simulink model "EqualizerSimulinkModel"  (R2025b)
settings: Solver=VariableStepAuto  StartTime=0.0  StopTime=10.0  RelTol=1e-3
undefined symbols (not defined in the file): dspblkCoreblockFVToolHelper, gcbh
libraries: simulink x5, dspvision x1

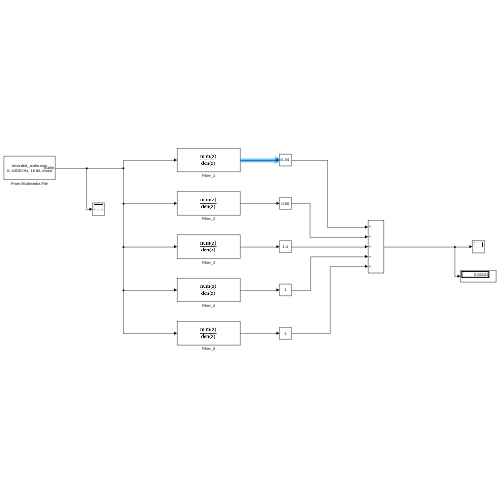
[thumbnail: Simulink's stored preview of the top-level diagram]
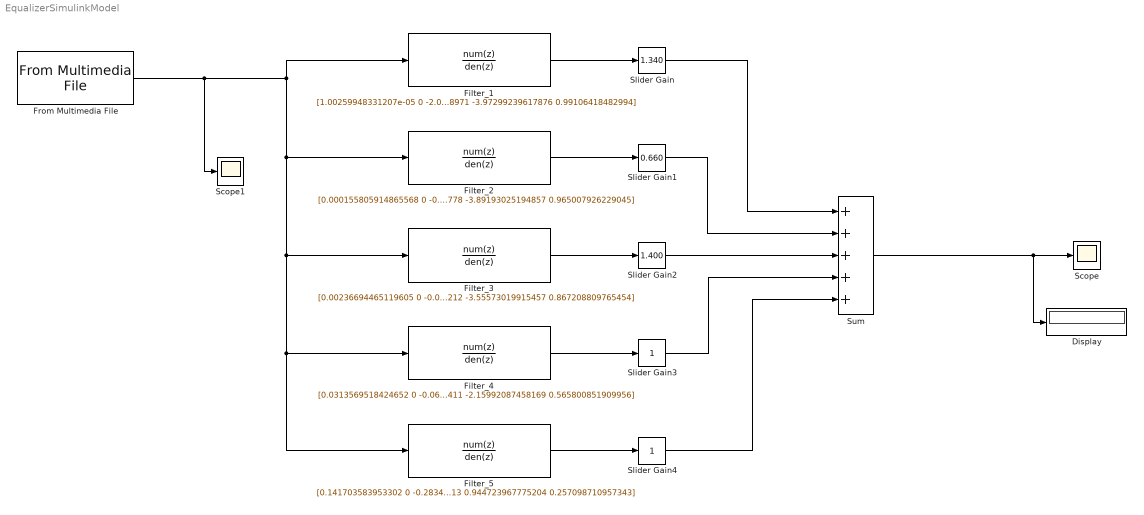
== system EqualizerSimulinkModel ==
  Display : Display
  Filter_1 : DiscreteTransferFcn  LoadFcn=dspblkCoreblockFVToolHelper(gcbh,'load');  Numerator=[1.00259948331207e-05 0 -2.00519896662413e-05 0 1.00259948331207e-05]  Denominator=[1 -3.99086330657876 5.97279152438971 -3.97299239617876 0.99106418482994]  SampleTime=2.2676e-05
      settings: CopyFcn=dspblkCoreblockFVToolHelper(gcbh,'copy');  DeleteFcn=dspblkCoreblockFVToolHelper(gcbh,'close');  ModelCloseFcn=dspblkCoreblockFVToolHelper(gcbh,'close');  PreSaveFcn=dspblkCoreblockFVToolHelper(gcbh,'presave');  PostSaveFcn=dspblkCoreblockFVToolHelper(gcbh,'postsave');  CloseFcn=dspblkCoreblockFVToolHelper(gcbh,'close');
  Filter_2 : DiscreteTransferFcn  Numerator=[0.000155805914865568 0 -0.000311611829731135 0 0.000155805914865568]  Denominator=[1 -3.96187000702167 5.88879391378778 -3.89193025194857 0.965007926229045]  SampleTime=2.2676e-05
  Filter_3 : DiscreteTransferFcn  Numerator=[0.00236694465119605 0 -0.0047338893023921 0 0.00236694465119605]  Denominator=[1 -3.81861928129895 5.50752375188212 -3.55573019915457 0.867208809765454]  SampleTime=2.2676e-05
  Filter_4 : DiscreteTransferFcn  Numerator=[0.0313569518424652 0 -0.0627139036849304 0 0.0313569518424652]  Denominator=[1 -2.88919382275762 3.56047322046411 -2.15992087458169 0.565800851909956]  SampleTime=2.2676e-05
  Filter_5 : DiscreteTransferFcn  Numerator=[0.141703583953302 0 -0.283407167906604 0 0.141703583953302]  Denominator=[1 2.11009924395369 1.88829530087313 0.944723967775204 0.257098710957343]  SampleTime=2.2676e-05
  From Multimedia File : dspvision/From Multimedia File  inputFilename=/MATLAB Drive/recorded_audio.wav  readRange=[1 Inf]  loop=on  numPlays=inf  outputStreams=Audio only  videoDataType=single  audioDataType=double  inheritSampleTime=on  userDefinedSampleTime=1/30  noAudioOutput=off  isIntensityVideo=off  fourcc=RGB  colorVideoFormat=One multidimensional signal  outputEOF=off  dataOrg=Column-major  audioFrameSize=1  computeAudioFrameSize=off  outSamplingMode=Sample based
      settings: LibrarySourceBlock=dspsrcs4/From Multimedia File
  Scope : Scope
      settings: ActiveDisplayYMinimum=-0.41885888280829847  ActiveDisplayYMaximum=0.33848681414686327
  Scope1 : Scope
      settings: ActiveDisplayYMinimum=-0.4656219482421875  ActiveDisplayYMaximum=0.5013275146484375
  Slider Gain : simulink/Math Operations/Slider Gain  gain=1.340  low=0  high=2
  Slider Gain1 : simulink/Math Operations/Slider Gain  gain=0.660  low=0  high=2
  Slider Gain2 : simulink/Math Operations/Slider Gain  gain=1.400  low=0  high=2
  Slider Gain3 : simulink/Math Operations/Slider Gain  gain=1  low=0  high=2
  Slider Gain4 : simulink/Math Operations/Slider Gain  gain=1  low=0  high=2
  Sum : Sum  Inputs=+++++
  wires:
  From Multimedia File/1 -> Scope1/1, Filter_5/1, Filter_4/1, Filter_3/1, Filter_2/1, Filter_1/1
  Sum/1 -> Display/1, Scope/1
  Filter_1/1 -> Slider Gain/1
  Filter_2/1 -> Slider Gain1/1
  Filter_3/1 -> Slider Gain2/1
  Filter_4/1 -> Slider Gain3/1
  Filter_5/1 -> Slider Gain4/1
  Slider Gain4/1 -> Sum/5
  Slider Gain3/1 -> Sum/4
  Slider Gain2/1 -> Sum/3
  Slider Gain1/1 -> Sum/2
  Slider Gain/1 -> Sum/1
